simulink model "test08"  (R2021a)
settings: Solver=VariableStepAuto  StartTime=0.0  StopTime=10  RelTol=1e-3
values from neighbouring files (symbols this model uses):
  crop_params = crop_p    [test08_script.m]
  x0_crop = crop_ic    [test08_script.m]
libraries: HORTISIM x15
(part 1 of 2)
settings Model: Creator=djoroya  LastModifiedBy=djoroya
settings DebuggingCC: UnconnectedInputMsg=none  UnconnectedOutputMsg=none  UnconnectedLineMsg=none

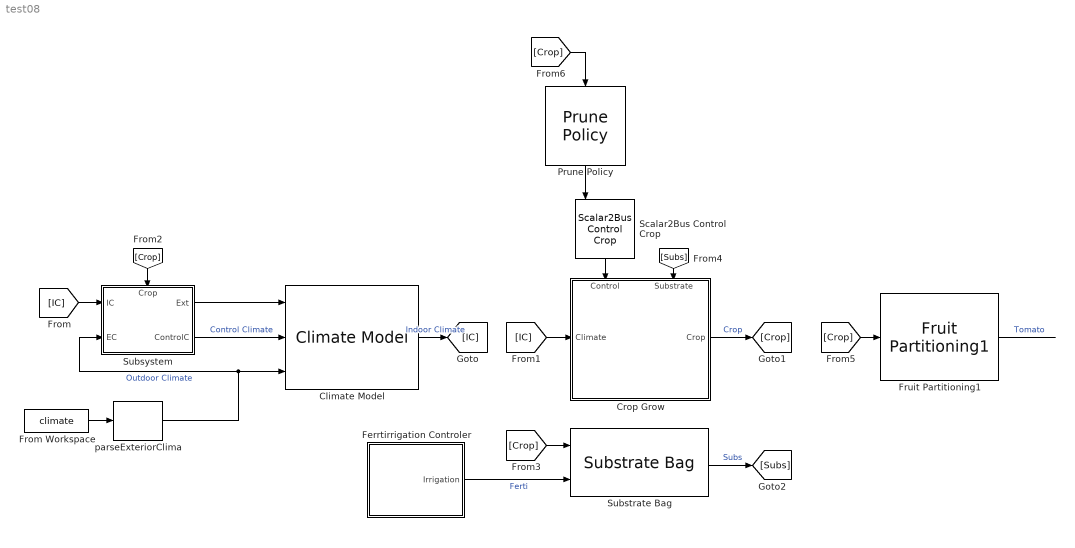
== system test08 ==
  Climate Model : HORTISIM/Climate/Models/Climate Model  params=params  x0=cic
      settings: SourceProductName=Horti Simulator
      mask Display: image('$imagefile'); % Use "Edit Image" on toolstrip to change.
  Crop Grow : Subsystem  AncestorBlock=HORTISIM/Horticulture/Models/Crop Grow  mask{params=crop_params, x0=x0_crop}
      settings: PortSchema="{\"entries\":[{\"content\":{\"sides\":[{\"content\":{\"connectorIds\":[\"In1\"]},\"type\":\"ConnectorPlacement.EquallySpacedRectSide\",\"uuid\":\"7d52d4c6-bc72-40ae-ba7a-fef791f60555\"},{\"content\":{\"connectorIds\":[\"Out1\"],\"side\":\"RIGHT\"},\"type\":\"ConnectorPlacement.EquallySpacedRectSide\",\"uuid\":\"3a9c2840-361d-4677-a7cc-c5f954b33f07\"},{\"content\":{\"connectorIds\":[\"In2\",\"In3\"],\"side\":\"TOP\"},\"type\":\"ConnectorPlacement.EquallySpacedRectSide\",\"uuid\":\"4fc8b0ee-86a8-4f1e-9fcc-25f95949aa32\"},{\"content\":{\"connectorIds\":[],\"side\":\"BOTTOM\"},\"type\":\"ConnectorPlacement.EquallySpacedRectSide\",\"uuid\":\"254dc665-acaf-49d5-9184-a028de083de6\"}]},\"type\":\"ConnectorPlacement.EquallySpacedConnector\",\"uuid\":\"4a2a8912-594b-41a4-9c04-2b6ae0329b55\"}],\"packageUris\":[\"http://schema.mathworks.com/mf0/Connector/R2020b\"],\"version\":\"1.0\"}"
      mask Display: image('$imagefile'); % Use "Edit Image" on toolstrip to change.
  Ferrtirrigation Controler : Subsystem  AncestorBlock="HORTISIM/Horticulture/Controls/Ferrtirrigation  Controler"
      mask Display: image('$imagefile'); % Use "Edit Image" on toolstrip to change.
  From Workspace : FromWorkspace  VariableName=climate
  Fruit Partitioning1 : HORTISIM/Horticulture/Models/Fruit Partitioning1  x0=x0_fruit  params=params_fruit
      settings: SourceProductName=Horti Simulator
      mask Display: image('tomato.png'); % Use "Edit Image" on toolstrip to change.
  Prune Policy : HORTISIM/Horticulture/Controls/Prune Policy  SystemSampleTime=-1  VariantActivationTime=update diagram  Latency=0  AutoFrameSizeCalculation=off
      settings: SourceProductName=Horti Simulator
      mask Display: image('$imagefile'); % Use "Edit Image" on toolstrip to change.
  Scalar2Bus Control Crop : HORTISIM/Other  Functions/Scalar2Bus Control Crop  SystemSampleTime=-1  VariantActivationTime=update diagram  Latency=0  AutoFrameSizeCalculation=off
      settings: SourceProductName=Horti Simulator
  Substrate Bag : HORTISIM/Horticulture/Models/Substrate Bag  x0=x0_substrate  params=substrate_params
      settings: SourceProductName=Horti Simulator
      mask Display: image('substrate.png'); % Use "Edit Image" on toolstrip to change.
  Subsystem : Subsystem
      settings: PortSchema="{\"entries\":[{\"content\":{\"sides\":[{\"content\":{\"connectorIds\":[\"In1\",\"In2\"]},\"type\":\"ConnectorPlacement.EquallySpacedRectSide\",\"uuid\":\"05a20284-31f0-4954-ac42-b08c051c723b\"},{\"content\":{\"connectorIds\":[\"Out1\",\"Out2\"],\"side\":\"RIGHT\"},\"type\":\"ConnectorPlacement.EquallySpacedRectSide\",\"uuid\":\"7e4ab434-6629-473e-82a5-f81f17f0ab6e\"},{\"content\":{\"connectorIds\":[\"In3\"],\"side\":\"TOP\"},\"type\":\"ConnectorPlacement.EquallySpacedRectSide\",\"uuid\":\"2ea64524-8947-456a-a977-2c05776eabaa\"}]},\"type\":\"ConnectorPlacement.EquallySpacedConnector\",\"uuid\":\"6035ded9-300f-4f3c-adde-f9d2e7ea6cf9\"}],\"packageUris\":[\"http://schema.mathworks.com/mf0/Connector/R2020b\"],\"version\":\"1.0\"}"
  parseExteriorClima : HORTISIM/Other  Functions/parseExteriorClima  SystemSampleTime=-1  VariantActivationTime=update diagram  Latency=0  AutoFrameSizeCalculation=off
      settings: SourceProductName=Horti Simulator
  wires:
  From Workspace/1 -> parseExteriorClima/1
  parseExteriorClima/1 -> Climate Model/3, Subsystem/2(EC)  "Outdoor Climate"
  Climate Model/1 -> [IC]  "Indoor Climate"
  Subsystem/2(ControlC) -> Climate Model/2  "Control Climate"
  [IC] -> Subsystem/1(IC)
  Subsystem/1(Ext) -> Climate Model/1
  [IC] -> Crop Grow/1(Climate)
  Crop Grow/1(Crop) -> [Crop]  "Crop"
  [Crop] -> Subsystem/3(Crop)
  [Crop] -> Substrate Bag/1
  Substrate Bag/1 -> [Subs]  "Subs"
  [Subs] -> Crop Grow/3(Substrate)
  Ferrtirrigation Controler/1(Irrigation) -> Substrate Bag/2  "Ferti"
  [Crop] -> Fruit Partitioning1/1
  Fruit Partitioning1/1 -> ?  "Tomato"
  Scalar2Bus Control Crop/1 -> Crop Grow/2(Control)
  Prune Policy/1 -> Scalar2Bus Control Crop/1
  [Crop] -> Prune Policy/1

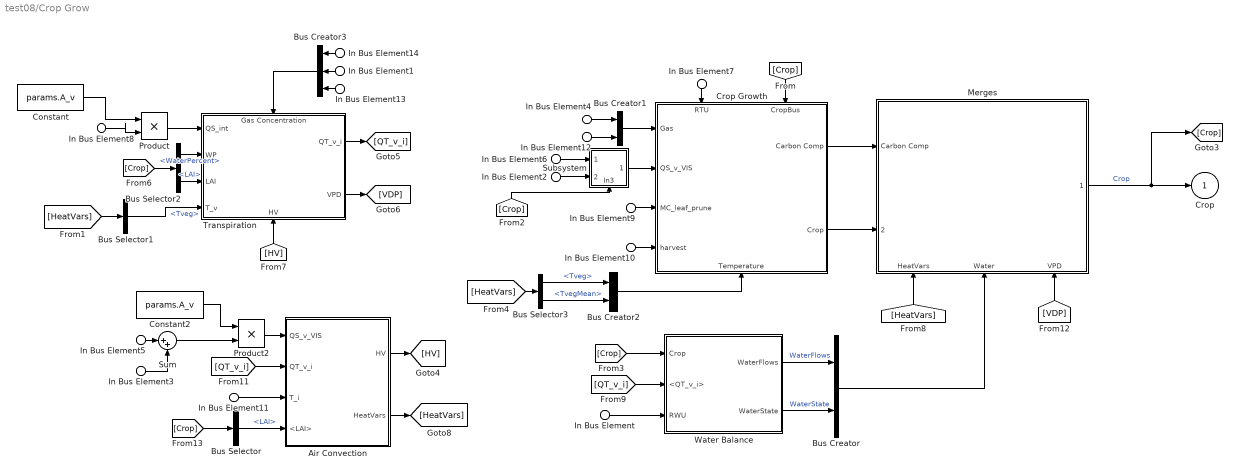
== system test08/Crop Grow ==
  In Bus Element8 : Inport  PortName=Climate  Element=QS.R_int
  In Bus Element3 : Inport  PortName=Climate  Element=QS.R_int
  In Bus Element2 : Inport  PortName=Climate  Element=QS.R_int
  In Bus Element11 : Inport  PortName=Climate  Element=Temp.Tair
  In Bus Element4 : Inport  PortName=Climate  Element=Gas.C_c
  In Bus Element12 : Inport  PortName=Climate  Element=Gas.rho_i
  In Bus Element13 : Inport  PortName=Climate  Element=Gas.rho_i
  In Bus Element1 : Inport  PortName=Climate  Element=Gas.C_c_ppm
  In Bus Element14 : Inport  PortName=Climate  Element=Gas.C_w
  In Bus Element9 : Inport  Port=2  PortName=Control  Element=Prune
  In Bus Element5 : Inport  Port=2  PortName=Control  Element=Artificial Rad
  In Bus Element6 : Inport  Port=2  PortName=Control  Element=Artificial Rad
  In Bus Element10 : Inport  Port=2  PortName=Control  Element=Harvest
  In Bus Element : Inport  Port=3  PortName=Substrate  Element=Uptake.Water
  In Bus Element7 : Inport  Port=3  PortName=Substrate  Element=Uptake.Nutrients
  Air Convection : Subsystem
  Bus Creator : BusCreator  Inputs=2
  Bus Creator1 : BusCreator  Inputs=2
  Bus Creator2 : BusCreator  Inputs=2
  Bus Creator3 : BusCreator  Inputs=3
  Bus Selector : BusSelector  OutputSignals=LAI
  Bus Selector1 : BusSelector  OutputSignals=Tveg
  Bus Selector2 : BusSelector  OutputSignals=WaterPercent,LAI
  Bus Selector3 : BusSelector  OutputSignals=Tveg,TvegMean
  Constant : Constant  Value=params.A_v
  Constant2 : Constant  Value=params.A_v
  Crop Growth : Subsystem
      settings: PortSchema="{\"entries\":[{\"content\":{\"sides\":[{\"content\":{\"connectorIds\":[\"In1\",\"In2\",\"In3\",\"In4\"]},\"type\":\"ConnectorPlacement.EquallySpacedRectSide\",\"uuid\":\"e694206d-cf53-43ea-b790-8b83ac78aa3a\"},{\"content\":{\"connectorIds\":[\"Out1\",\"Out2\"],\"side\":\"RIGHT\"},\"type\":\"ConnectorPlacement.EquallySpacedRectSide\",\"uuid\":\"93817abb-865a-4529-a53b-9aa59cd1156c\"},{\"content\":{\"connectorIds\":[\"In5\",\"In6\"],\"side\":\"TOP\"},\"type\":\"ConnectorPlacement.EquallySpacedRectSide\",\"uuid\":\"edd59083-b991-4826-870e-7da3bc3e48d4\"},{\"content\":{\"connectorIds\":[\"In7\"],\"side\":\"BOTTOM\"},\"type\":\"ConnectorPlacement.EquallySpacedRectSide\",\"uuid\":\"aa2b3153-bf16-47ed-b19e-45b92f713263\"}]},\"type\":\"ConnectorPlacement.EquallySpacedConnector\",\"uuid\":\"72640b1e-82d8-4725-bb34-7435bfc9f969\"}],\"packageUris\":[\"http://schema.mathworks.com/mf0/Connector/R2020b\"],\"version\":\"1.0\"}"
  Merges : Subsystem
      settings: PortSchema="{\"entries\":[{\"content\":{\"sides\":[{\"content\":{\"connectorIds\":[\"In1\",\"In2\"]},\"type\":\"ConnectorPlacement.EquallySpacedRectSide\",\"uuid\":\"f4887da6-2928-4f39-8f5f-a84d343119b4\"},{\"content\":{\"connectorIds\":[\"Out1\"],\"side\":\"RIGHT\"},\"type\":\"ConnectorPlacement.EquallySpacedRectSide\",\"uuid\":\"0df0d8c4-f19c-45da-a42d-26f0e872c274\"},{\"content\":{\"connectorIds\":[],\"side\":\"TOP\"},\"type\":\"ConnectorPlacement.EquallySpacedRectSide\",\"uuid\":\"3b0cc3f6-1cfb-43ac-8908-74a7a76931e3\"},{\"content\":{\"connectorIds\":[\"In3\",\"In4\",\"In5\"],\"side\":\"BOTTOM\"},\"type\":\"ConnectorPlacement.EquallySpacedRectSide\",\"uuid\":\"7e6672ca-68aa-4c3f-955a-240d8575a2c6\"}]},\"type\":\"ConnectorPlacement.EquallySpacedConnector\",\"uuid\":\"a8299565-1b25-4490-849f-a8fa281592c1\"}],\"packageUris\":[\"http://schema.mathworks.com/mf0/Connector/R2020b\"],\"version\":\"1.0\"}"
  Product : Product
  Product2 : Product
  Subsystem : Subsystem
      settings: PortSchema="{\"entries\":[{\"content\":{\"sides\":[{\"content\":{\"connectorIds\":[\"In1\",\"In2\"]},\"type\":\"ConnectorPlacement.EquallySpacedRectSide\",\"uuid\":\"c9e251e2-f19d-4856-b15c-3b9f1eb64f83\"},{\"content\":{\"connectorIds\":[\"Out1\"],\"side\":\"RIGHT\"},\"type\":\"ConnectorPlacement.EquallySpacedRectSide\",\"uuid\":\"10734817-c937-42fb-8ae5-9505620c6f0f\"},{\"content\":{\"connectorIds\":[],\"side\":\"TOP\"},\"type\":\"ConnectorPlacement.EquallySpacedRectSide\",\"uuid\":\"8c056440-d8bf-4ff4-85aa-0f6a5eb7f23f\"},{\"content\":{\"connectorIds\":[\"In3\"],\"side\":\"BOTTOM\"},\"type\":\"ConnectorPlacement.EquallySpacedRectSide\",\"uuid\":\"dd07dcd8-5298-4126-bdbb-0b047f66f0f4\"}]},\"type\":\"ConnectorPlacement.EquallySpacedConnector\",\"uuid\":\"13e72cfa-9d8f-4756-adac-f24fb0238c2a\"}],\"packageUris\":[\"http://schema.mathworks.com/mf0/Connector/R2020b\"],\"version\":\"1.0\"}"
  Sum : Sum  Inputs=|++
  Transpiration : Subsystem
      settings: PortSchema="{\"entries\":[{\"content\":{\"sides\":[{\"content\":{\"connectorIds\":[\"In1\",\"In2\",\"In3\",\"In4\"]},\"type\":\"ConnectorPlacement.EquallySpacedRectSide\",\"uuid\":\"d6bbd0cc-329a-44d5-b58b-a93078f7e5d1\"},{\"content\":{\"connectorIds\":[\"Out1\",\"Out2\"],\"side\":\"RIGHT\"},\"type\":\"ConnectorPlacement.EquallySpacedRectSide\",\"uuid\":\"249abf44-6c9b-4b00-a2f9-2043ee582e13\"},{\"content\":{\"connectorIds\":[\"In5\"],\"side\":\"TOP\"},\"type\":\"ConnectorPlacement.EquallySpacedRectSide\",\"uuid\":\"efa2d349-63e9-4701-9d30-a0c2adbee945\"},{\"content\":{\"connectorIds\":[\"In6\"],\"side\":\"BOTTOM\"},\"type\":\"ConnectorPlacement.EquallySpacedRectSide\",\"uuid\":\"decf1794-1744-434d-adf6-c7060d48f04b\"}]},\"type\":\"ConnectorPlacement.EquallySpacedConnector\",\"uuid\":\"1e3e15aa-c080-4684-9da5-24f03928e17f\"}],\"packageUris\":[\"http://schema.mathworks.com/mf0/Connector/R2020b\"],\"version\":\"1.0\"}"
  Water Balance : Subsystem
  Crop : Outport
  wires:
  [Crop] -> Subsystem/3(In3)
  In Bus Element10/1 -> Crop Growth/4(harvest)
  In Bus Element/1 -> Water Balance/3(RWU)
  Bus Selector3/1 -> Bus Creator2/1  "<Tveg>"
  [HeatVars] -> Bus Selector3/1
  [HeatVars] -> Bus Selector1/1
  Bus Creator/1 -> Merges/4(Water)
  Water Balance/2(WaterState) -> Bus Creator/2  "WaterState"
  Water Balance/1(WaterFlows) -> Bus Creator/1  "WaterFlows"
  In Bus Element7/1 -> Crop Growth/5(RTU)
  Subsystem/1(Out1) -> Crop Growth/2(QS_v_VIS)
  In Bus Element2/1 -> Subsystem/2(In2)
  In Bus Element6/1 -> Subsystem/1(In1)
  Sum/1 -> Product2/2
  In Bus Element3/1 -> Sum/2
  In Bus Element5/1 -> Sum/1
  Constant2/1 -> Product2/1
  Product2/1 -> Air Convection/1(QS_v_VIS)
  Product/1 -> Transpiration/1(QS_int)
  In Bus Element8/1 -> Product/2
  Constant/1 -> Product/1
  In Bus Element13/1 -> Bus Creator3/3
  In Bus Element1/1 -> Bus Creator3/2
  In Bus Element14/1 -> Bus Creator3/1
  [Crop] -> Crop Growth/6(CropBus)
  Air Convection/2(HeatVars) -> [HeatVars]
  Air Convection/1(HV) -> [HV]
  Bus Selector/1 -> Air Convection/4(<LAI>)  "<LAI>"
  In Bus Element11/1 -> Air Convection/3(T_i)
  [QT_v_i] -> Air Convection/2(QT_v_i)
  [QT_v_i] -> Water Balance/2(<QT_v_i>)
  [Crop] -> Water Balance/1(Crop)
  Crop Growth/2(Crop) -> Merges/2(" ")
  Crop Growth/1("Carbon Comp   ") -> Merges/1("Carbon Comp   ")
  Bus Creator2/1 -> Crop Growth/7(Temperature)
  In Bus Element9/1 -> Crop Growth/3(MC_leaf_prune)
  Bus Creator1/1 -> Crop Growth/1(Gas)
  [HeatVars] -> Merges/3(HeatVars)
  Bus Selector1/1 -> Transpiration/4(T_v)  "<Tveg>"
  [Crop] -> Bus Selector/1
  [VDP] -> Merges/5(VPD)
  Transpiration/2(VPD) -> [VDP]
  Transpiration/1(QT_v_i) -> [QT_v_i]
  Bus Selector2/2 -> Transpiration/3(LAI)  "<LAI>"
  [Crop] -> Bus Selector2/1
  Bus Selector2/1 -> Transpiration/2(WP)  "<WaterPercent>"
  Bus Creator3/1 -> Transpiration/5(Gas Concentration)
  [HV] -> Transpiration/6(HV)
  Bus Selector3/2 -> Bus Creator2/2  "<TvegMean>"
  In Bus Element12/1 -> Bus Creator1/2
  In Bus Element4/1 -> Bus Creator1/1
  Merges/1("    ") -> [Crop], Crop/1  "Crop"

== system test08/Ferrtirrigation Controler ==
  note: $kg\{H_2O\}/(s\cdot plant)$
  Bus Creator : BusCreator  Inputs=3  OutDataTypeStr=Bus: FLOW  NonVirtualBus=on
  Irrigation Controler : Subsystem
  "[Kelvin]" : Constant  Value=273.15 + 10
  kg/m^3 : Constant  Value=0.1 +zeros(8,1)
  Irrigation : Outport
  wires:
  kg/m^3/1 -> Bus Creator/3  "X"
  Irrigation Controler/1(Irrigation) -> Bus Creator/1  "f"
  "[Kelvin]"/1 -> Bus Creator/2  "T"
  Bus Creator/1 -> Irrigation/1

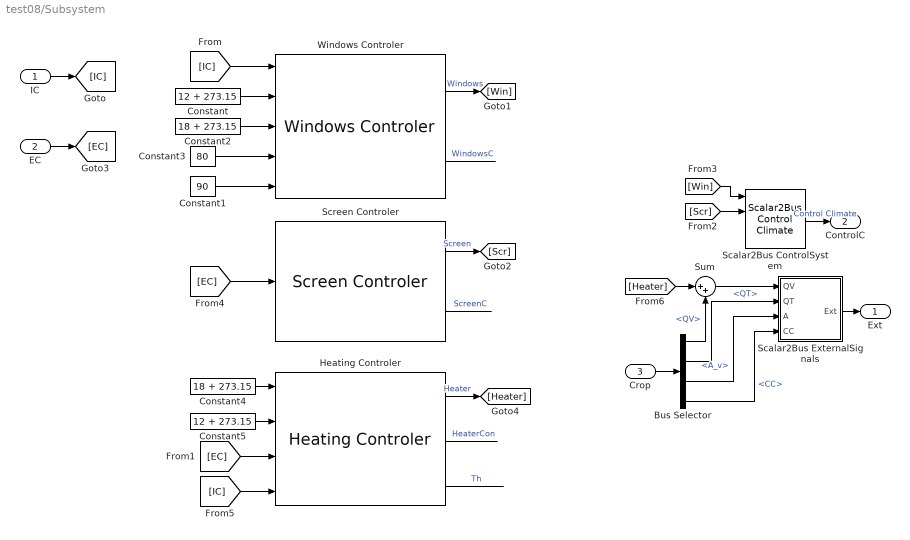
== system test08/Subsystem ==
  IC : Inport
  EC : Inport  Port=2
  Crop : Inport  Port=3
  Bus Selector : BusSelector  OutputSignals=HeatVars.QV,HeatVars.QT,A_v,CC
  Constant : Constant  Value=12 + 273.15
  Constant1 : Constant  Value=90
  Constant2 : Constant  Value=18 + 273.15
  Constant3 : Constant  Value=80
  Constant4 : Constant  Value=18 + 273.15
  Constant5 : Constant  Value=12 + 273.15
  Heating Controler : HORTISIM/Climate/Controls/Heating Controler  params=heat_p  x0=heat_ic
      settings: SourceProductName=Horti Simulator
  Scalar2Bus ControlSystem : HORTISIM/Other  Functions/Scalar2Bus  Control Climate  SystemSampleTime=-1  VariantActivationTime=update diagram  Latency=0  AutoFrameSizeCalculation=off
      settings: SourceProductName=Horti Simulator
  Scalar2Bus ExternalSignals : Subsystem
  Screen Controler : HORTISIM/Climate/Controls/Screen Controler  params=scr_p
      settings: SourceProductName=Horti Simulator
  Sum : Sum  Inputs=|++
  Windows Controler : HORTISIM/Climate/Controls/Windows Controler  params=win_p
      settings: SourceProductName=Horti Simulator
  Ext : Outport
  ControlC : Outport  Port=2
  wires:
  Constant2/1 -> Windows Controler/3
  Constant3/1 -> Windows Controler/4
  Windows Controler/2 -> ?  "WindowsC"
  Constant1/1 -> Windows Controler/5
  Constant/1 -> Windows Controler/2
  IC/1 -> [IC]
  [IC] -> Windows Controler/1
  Windows Controler/1 -> [Win]  "Windows"
  Screen Controler/1 -> [Scr]  "Screen"
  [Scr] -> Scalar2Bus ControlSystem/2
  [Win] -> Scalar2Bus ControlSystem/1
  Scalar2Bus ControlSystem/1 -> ControlC/1  "Control Climate"
  EC/1 -> [EC]
  [EC] -> Screen Controler/1
  Screen Controler/2 -> ?  "ScreenC"
  [EC] -> Heating Controler/3
  [IC] -> Heating Controler/4
  Constant4/1 -> Heating Controler/1
  Constant5/1 -> Heating Controler/2
  Heating Controler/1 -> [Heater]  "Heater"
  Scalar2Bus ExternalSignals/1(Ext) -> Ext/1
  Heating Controler/3 -> ?  "Th"
  Heating Controler/2 -> ?  "HeaterCon"
  Crop/1 -> Bus Selector/1
  Bus Selector/2 -> Scalar2Bus ExternalSignals/2(QT)  "<QT>"
  [Heater] -> Sum/1
  Sum/1 -> Scalar2Bus ExternalSignals/1(QV)
  Bus Selector/1 -> Sum/2  "<QV>"
  Bus Selector/3 -> Scalar2Bus ExternalSignals/3(A)  "<A_v>"
  Bus Selector/4 -> Scalar2Bus ExternalSignals/4(CC)  "<CC>"

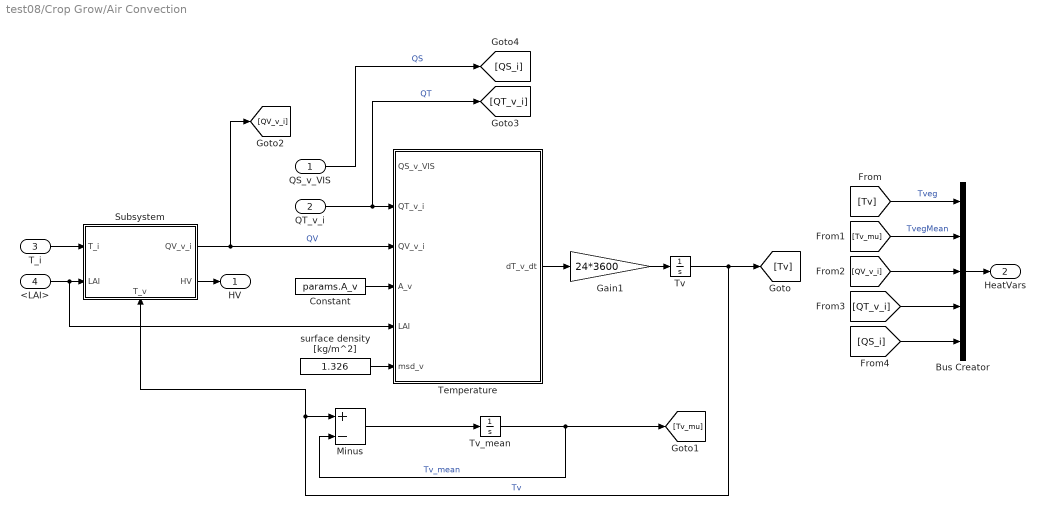
== system test08/Crop Grow/Air Convection ==
  QS_v_VIS : Inport
  QT_v_i : Inport  Port=2
  T_i : Inport  Port=3
  <LAI> : Inport  Port=4
  " Temperature" : MATLAB Function  TreatAsAtomicUnit=on
  Bus Creator : BusCreator  Inputs=5
  Constant : Constant  Value=params.A_v
  Gain1 : Gain  Gain=24*3600
  Minus : Sum  Inputs=+-
  Subsystem : Subsystem
      settings: PortSchema="{\"entries\":[{\"content\":{\"sides\":[{\"content\":{\"connectorIds\":[\"In1\",\"In2\"]},\"type\":\"ConnectorPlacement.EquallySpacedRectSide\",\"uuid\":\"4a223777-4148-4e71-aff8-25d93471e208\"},{\"content\":{\"connectorIds\":[\"Out1\",\"Out2\"],\"side\":\"RIGHT\"},\"type\":\"ConnectorPlacement.EquallySpacedRectSide\",\"uuid\":\"f67a472e-d82a-4194-8a1d-cf4d17d79652\"},{\"content\":{\"connectorIds\":[],\"side\":\"TOP\"},\"type\":\"ConnectorPlacement.EquallySpacedRectSide\",\"uuid\":\"dc13fded-a670-4e66-896d-6b985aeea447\"},{\"content\":{\"connectorIds\":[\"In3\"],\"side\":\"BOTTOM\"},\"type\":\"ConnectorPlacement.EquallySpacedRectSide\",\"uuid\":\"546dc1d6-9e48-4e4a-b9dc-c8e8ff8af02b\"}]},\"type\":\"ConnectorPlacement.EquallySpacedConnector\",\"uuid\":\"dd1fea49-cd8b-49b4-879c-c05a742382b3\"}],\"packageUris\":[\"http://schema.mathworks.com/mf0/Connector/R2020b\"],\"version\":\"1.0\"}"
  Tv : Integrator  InitialCondition=x0.Tv  AbsoluteTolerance=0.01
  Tv_mean : Integrator  InitialCondition=x0.Tv  AbsoluteTolerance=1e-3
  surface density [kg/m^2] : Constant  Value=1.326
  HV : Outport
  HeatVars : Outport  Port=2
  wires:
  Bus Creator/1 -> HeatVars/1
  [QS_i] -> Bus Creator/5
  [QT_v_i] -> Bus Creator/4
  [QV_v_i] -> Bus Creator/3
  [Tv_mu] -> Bus Creator/2  "TvegMean"
  [Tv] -> Bus Creator/1  "Tveg"
  QT_v_i/1 -> " Temperature"/2(QT_v_i), [QT_v_i]  "QT"
  QS_v_VIS/1 -> [QS_i]  "QS"
  Subsystem/1(QV_v_i) -> " Temperature"/3(QV_v_i), [QV_v_i]  "QV"
  Tv/1 -> Subsystem/3(T_v), Minus/1, [Tv]  "Tv"
  Minus/1 -> Tv_mean/1
  Tv_mean/1 -> Minus/2, [Tv_mu]  "Tv_mean"
  T_i/1 -> Subsystem/1(T_i)
  Subsystem/2(HV) -> HV/1
  <LAI>/1 -> " Temperature"/5(LAI), Subsystem/2(LAI)
  Constant/1 -> " Temperature"/4(A_v)
  surface density [kg/m^2]/1 -> " Temperature"/6(msd_v)
  " Temperature"/1(dT_v_dt) -> Gain1/1
  Gain1/1 -> Tv/1

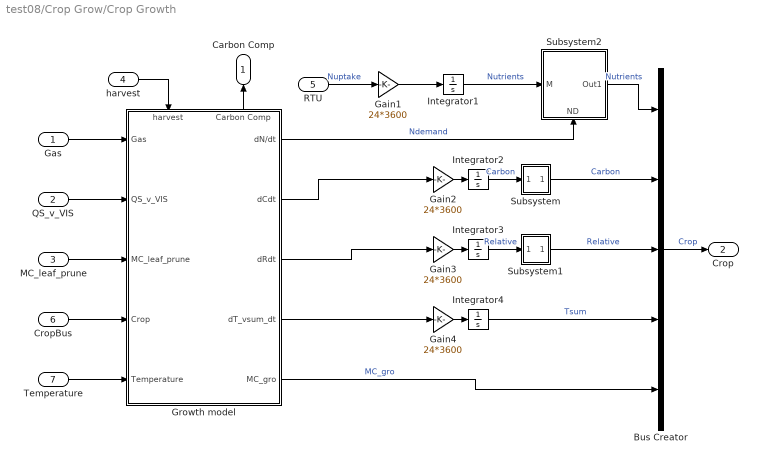
== system test08/Crop Grow/Crop Growth ==
  Gas : Inport
  QS_v_VIS : Inport  Port=2
  MC_leaf_prune : Inport  Port=3
  harvest : Inport  Port=4
  RTU : Inport  Port=5
  CropBus : Inport  Port=6
  Temperature : Inport  Port=7
  Bus Creator : BusCreator  Inputs=5
  Gain{1..4} (4 alike) : Gain  Gain=24*3600
  Growth model : Subsystem
      settings: PortSchema="{\"entries\":[{\"content\":{\"sides\":[{\"content\":{\"connectorIds\":[\"In1\",\"In2\",\"In3\",\"In4\",\"In5\"]},\"type\":\"ConnectorPlacement.EquallySpacedRectSide\",\"uuid\":\"524d3e03-5719-41db-bf49-dcf5dd5869ab\"},{\"content\":{\"connectorIds\":[\"Out1\",\"Out2\",\"Out3\",\"Out4\",\"Out5\"],\"side\":\"RIGHT\"},\"type\":\"ConnectorPlacement.EquallySpacedRectSide\",\"uuid\":\"b6ee0c40-6a76-4355-a893-3d13d29f29ea\"},{\"content\":{\"connectorIds\":[\"In6\",\"Out6\"],\"side\":\"TOP\"},\"type\":\"ConnectorPlacement.EquallySpacedRectSide\",\"uuid\":\"3cb45a24-0889-4a9a-ac04-e1ca208b77ae\"}]},\"type\":\"ConnectorPlacement.EquallySpacedConnector\",\"uuid\":\"fab17374-053c-4d8a-b11b-d7cd69978ad8\"}],\"packageUris\":[\"http://schema.mathworks.com/mf0/Connector/R2020b\"],\"version\":\"1.0\"}"
  Integrator1 : Integrator  InitialCondition=x0.N  AbsoluteTolerance=1e-4
  Integrator2 : Integrator  InitialCondition=x0.C  AbsoluteTolerance=1e-4
  Integrator3 : Integrator  InitialCondition=x0.R  AbsoluteTolerance=1e-9
  Integrator4 : Integrator  InitialCondition=x0.Tsum
  Subsystem : Subsystem
  Subsystem1 : Subsystem
  Subsystem2 : Subsystem
      settings: PortSchema="{\"entries\":[{\"content\":{\"sides\":[{\"content\":{\"connectorIds\":[\"In1\"]},\"type\":\"ConnectorPlacement.EquallySpacedRectSide\",\"uuid\":\"1f0226fa-6d14-4434-a5d5-098a94c6aa33\"},{\"content\":{\"connectorIds\":[\"Out1\"],\"side\":\"RIGHT\"},\"type\":\"ConnectorPlacement.EquallySpacedRectSide\",\"uuid\":\"12e08114-9d71-45f9-bd21-e03815fbba92\"},{\"content\":{\"connectorIds\":[],\"side\":\"TOP\"},\"type\":\"ConnectorPlacement.EquallySpacedRectSide\",\"uuid\":\"f70b570c-09d2-427a-8272-34c6eabee9a4\"},{\"content\":{\"connectorIds\":[\"In2\"],\"side\":\"BOTTOM\"},\"type\":\"ConnectorPlacement.EquallySpacedRectSide\",\"uuid\":\"db0772f6-92fe-46fe-85e5-ff48d92542ad\"}]},\"type\":\"ConnectorPlacement.EquallySpacedConnector\",\"uuid\":\"23ce1bc9-4d09-4c56-8e1c-5e49b0ef0462\"}],\"packageUris\":[\"http://schema.mathworks.com/mf0/Connector/R2020b\"],\"version\":\"1.0\"}"
  "Carbon Comp   " : Outport
  Crop : Outport  Port=2
  wires:
  harvest/1 -> Growth model/6(harvest)
  Growth model/1(dN/dt) -> Subsystem2/2(ND)  "Ndemand"
  Subsystem2/1(Out1) -> Bus Creator/1  "Nutrients"
  Integrator1/1 -> Subsystem2/1(M)  "Nutrients"
  RTU/1 -> Gain1/1  "Nuptake"
  Gain1/1 -> Integrator1/1
  Subsystem1/1(Out1) -> Bus Creator/3  "Relative"
  Integrator3/1 -> Subsystem1/1(In1)  "Relative"
  Integrator2/1 -> Subsystem/1(In1)  "Carbon"
  Subsystem/1(Out1) -> Bus Creator/2  "Carbon"
  Growth model/5(MC_gro) -> Bus Creator/5  "MC_gro"
  Temperature/1 -> Growth model/5(Temperature)
  CropBus/1 -> Growth model/4(Crop)
  Gain2/1 -> Integrator2/1
  QS_v_VIS/1 -> Growth model/2(QS_v_VIS)
  Growth model/2(dCdt) -> Gain2/1
  Growth model/4(dT_vsum_dt) -> Gain4/1
  Gain4/1 -> Integrator4/1
  Gain3/1 -> Integrator3/1
  Gas/1 -> Growth model/1(Gas)
  Growth model/3(dRdt) -> Gain3/1
  Integrator4/1 -> Bus Creator/4  "Tsum"
  MC_leaf_prune/1 -> Growth model/3(MC_leaf_prune)
  Growth model/6("Carbon Comp   ") -> "Carbon Comp   "/1
  Bus Creator/1 -> Crop/1  "Crop"

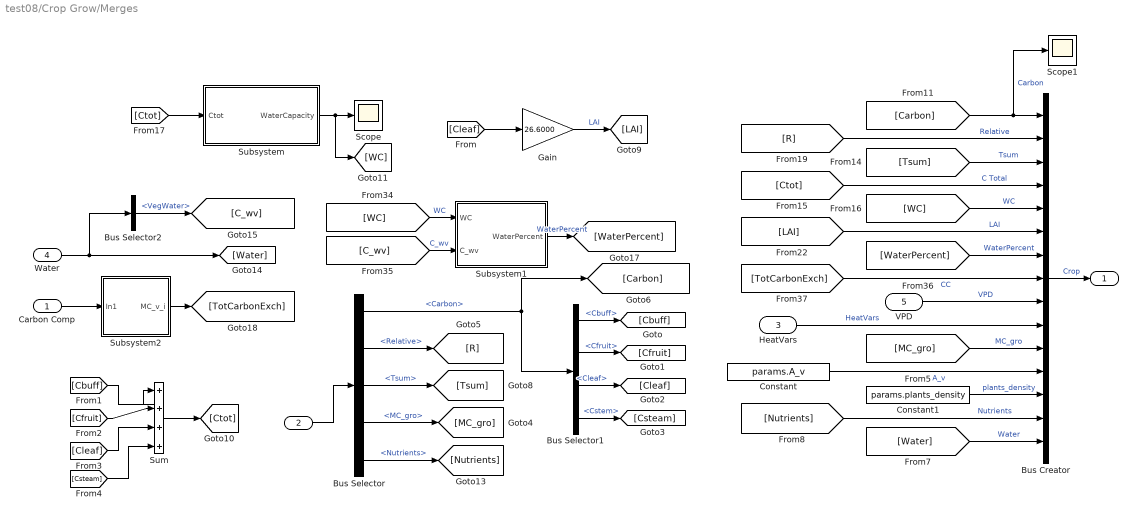
== system test08/Crop Grow/Merges ==
  "Carbon Comp   " : Inport
  " " : Inport  Port=2
  HeatVars : Inport  Port=3
  Water : Inport  Port=4
  VPD : Inport  Port=5
  Bus Creator : BusCreator  Inputs=15
  Bus Selector : BusSelector  OutputSignals=Carbon,Relative,Tsum,MC_gro,Nutrients
  Bus Selector1 : BusSelector  OutputSignals=Cbuff,Cfruit,Cleaf,Cstem
  Bus Selector2 : BusSelector  OutputSignals=WaterState.VegWater
  Constant : Constant  Value=params.A_v
  Constant1 : Constant  Value=params.plants_density
  Gain : Gain  Gain=26.6000
  Scope : Scope
  Scope1 : Scope
  Subsystem : Subsystem
  Subsystem1 : Subsystem
  Subsystem2 : Subsystem
  Sum : Sum  Inputs=|++++
  "    " : Outport
  wires:
  [Nutrients] -> Bus Creator/14  "Nutrients"
  Bus Selector/5 -> [Nutrients]  "<Nutrients>"
  Constant1/1 -> Bus Creator/13  "plants_density"
  [Ctot] -> Bus Creator/4  "C Total"
  Subsystem2/1(MC_v_i) -> [TotCarbonExch]
  [C_wv] -> Subsystem1/2(C_wv)  "C_wv"
  Bus Selector2/1 -> [C_wv]  "<VegWater>"
  Bus Selector/2 -> [R]  "<Relative>"
  Bus Selector1/2 -> [Cfruit]  "<Cfruit>"
  "Carbon Comp   "/1 -> Subsystem2/1(In1)
  Bus Selector/3 -> [Tsum]  "<Tsum>"
  [Carbon] -> Bus Creator/1, Scope1/1  "Carbon"
  [Water] -> Bus Creator/15  "Water"
  [WaterPercent] -> Bus Creator/7  "WaterPercent"
  Constant/1 -> Bus Creator/12  "A_v"
  [Csteam] -> Sum/4
  HeatVars/1 -> Bus Creator/10  "HeatVars"
  [MC_gro] -> Bus Creator/11  "MC_gro"
  Bus Selector/4 -> [MC_gro]  "<MC_gro>"
  [WC] -> Bus Creator/5  "WC"
  VPD/1 -> Bus Creator/9  "VPD"
  [TotCarbonExch] -> Bus Creator/8  "CC"
  Subsystem1/1(WaterPercent) -> [WaterPercent]  "WaterPercent"
  [WC] -> Subsystem1/1(WC)  "WC"
  Bus Selector1/4 -> [Csteam]  "<Cstem>"
  Bus Creator/1 -> "    "/1  "Crop"
  Bus Selector1/3 -> [Cleaf]  "<Cleaf>"
  Bus Selector1/1 -> [Cbuff]  "<Cbuff>"
  " "/1 -> Bus Selector/1
  [R] -> Bus Creator/2  "Relative"
  [LAI] -> Bus Creator/6  "LAI"
  [Tsum] -> Bus Creator/3  "Tsum"
  Water/1 -> [Water], Bus Selector2/1
  Bus Selector/1 -> [Carbon], Bus Selector1/1  "<Carbon>"
  Sum/1 -> [Ctot]
  [Cleaf] -> Sum/3
  [Cfruit] -> Sum/2
  [Cbuff] -> Sum/1
  [Ctot] -> Subsystem/1(Ctot)
  Subsystem/1(WaterCapacity) -> Scope/1, [WC]
  Gain/1 -> [LAI]  "LAI"
  [Cleaf] -> Gain/1

== system test08/Crop Grow/Subsystem ==
  In1 : Inport
  In2 : Inport  Port=2
  In3 : Inport  Port=3
  Bus Selector : BusSelector  OutputSignals=LAI
  Constant1 : Constant  Value=params.A_v
  Gain : Gain  Gain=2
  Product1 : Product  Inputs=3
  Scope : Scope
  Scope1 : Scope
  Subsystem : Subsystem
  Subsystem1 : Subsystem
  Sum : Sum  Inputs=|++
  Sum1 : Sum  Inputs=|++
  Out1 : Outport
  wires:
  Gain/1 -> Out1/1
  Product1/1 -> Gain/1
  Sum/1 -> Product1/1, Scope1/1
  [a_v_fVIS] -> Sum/2
  [a_v_rVIS] -> Sum/1
  Subsystem1/1(Out1) -> [a_v_rVIS]
  Bus Selector/1 -> Subsystem/1(<LAI>), Subsystem1/1(<LAI>)  "<LAI>"
  Subsystem/1(Out1) -> [a_v_fVIS], Scope/1
  In3/1 -> Bus Selector/1
  Constant1/1 -> Product1/2
  In1/1 -> Sum1/1
  Sum1/1 -> Product1/3
  In2/1 -> Sum1/2

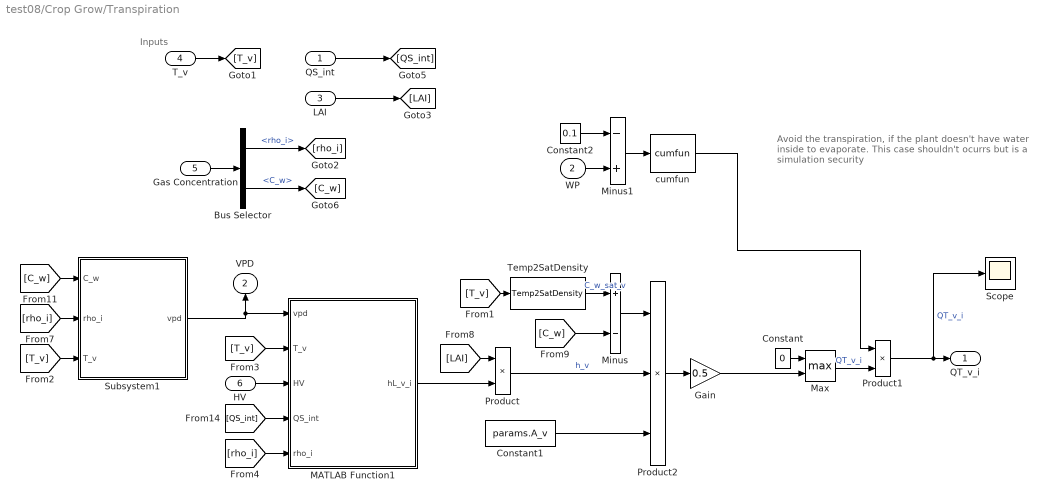
== system test08/Crop Grow/Transpiration ==
  note: Inputs
  note: Avoid the transpiration, if the plant
      |  doesn't have water inside to evaporate.
      | This case shouldn't ocurrs but is a simulation security
  QS_int : Inport
  WP : Inport  Port=2
  LAI : Inport  Port=3
  T_v : Inport  Port=4
  Gas Concentration : Inport  Port=5
  HV : Inport  Port=6
  Bus Selector : BusSelector  OutputSignals=rho_i,C_w
  Constant : Constant  Value=0
  Constant1 : Constant  Value=params.A_v
  Constant2 : Constant  Value=0.1
  Gain : Gain  Gain=0.5
  MATLAB Function1 : MATLAB Function  TreatAsAtomicUnit=on
  Max : MinMax  Function=max  Inputs=2
  Minus : Sum  Inputs=+-
  Minus1 : Sum  Inputs=-+
  Product : Product
  Product1 : Product
  Product2 : Product  Inputs=3
  Scope : Scope
  Subsystem1 : Subsystem
  Temp2SatDensity : HORTISIM/Other  Functions/Temp2SatDensity  SystemSampleTime=-1  VariantActivationTime=update diagram  Latency=0  AutoFrameSizeCalculation=off
      settings: SourceProductName=Horti Simulator
  cumfun : HORTISIM/Other  Functions/cumfun  SystemSampleTime=-1  VariantActivationTime=update diagram  Latency=0  AutoFrameSizeCalculation=off
      settings: SourceProductName=Horti Simulator
  QT_v_i : Outport
  VPD : Outport  Port=2
  wires:
  Minus1/1 -> cumfun/1
  cumfun/1 -> Product1/1
  Constant2/1 -> Minus1/1
  WP/1 -> Minus1/2
  [rho_i] -> MATLAB Function1/5(rho_i)
  [T_v] -> MATLAB Function1/2(T_v)
  Subsystem1/1(vpd) -> MATLAB Function1/1(vpd), VPD/1
  HV/1 -> MATLAB Function1/3(HV)
  [QS_int] -> MATLAB Function1/4(QS_int)
  MATLAB Function1/1(hL_v_i) -> Product/2
  [LAI] -> Product/1
  LAI/1 -> [LAI]
  [T_v] -> Subsystem1/3(T_v)
  [rho_i] -> Subsystem1/2(rho_i)
  [C_w] -> Subsystem1/1(C_w)
  Temp2SatDensity/1 -> Minus/1  "C_w_sat_v"
  [T_v] -> Temp2SatDensity/1
  Bus Selector/2 -> [C_w]  "<C_w>"
  Bus Selector/1 -> [rho_i]  "<rho_i>"
  Gas Concentration/1 -> Bus Selector/1
  QS_int/1 -> [QS_int]
  T_v/1 -> [T_v]
  [C_w] -> Minus/2
  Minus/1 -> Product2/1
  Product/1 -> Product2/2  "h_v"
  Constant1/1 -> Product2/3
  Product2/1 -> Gain/1
  Product1/1 -> QT_v_i/1, Scope/1  "QT_v_i"
  Constant/1 -> Max/1
  Max/1 -> Product1/2  "QT_v_i"
  Gain/1 -> Max/2

== system test08/Crop Grow/Water Balance ==
  note: $kg\{H_2O\}/(s\cdot m^2)$
  note: $kg\{H_2O\}/m^2$
  note: $kg\{H_2O\}/(s\cdot m^2)$
  Crop : Inport
  <QT_v_i> : Inport  Port=2
  RWU : Inport  Port=3
  Bus Selector : BusSelector  OutputSignals=WaterPercent,WC,A_v
  Divide : Product  Inputs=*//
  H_fg : Constant  Value=2437000
  Subsystem : Subsystem
  Subsystem1 : Subsystem
  Out Bus Element : Outport  PortName=WaterFlows  Element=WaterDemand
  Out Bus Element1 : Outport  PortName=WaterFlows  Element=WaterUptake
  Out Bus Element3 : Outport  PortName=WaterFlows  Element=MW_QT
  Out Bus Element6 : Outport  Port=2  PortName=WaterState  Element=VegWater
  wires:
  [MW_QT] -> Out Bus Element3/1
  Subsystem/1(C_wv) -> Out Bus Element6/1
  RWU/1 -> Subsystem/1(Real Water Uptake), [RWU]  "Real Water Uptake"
  Subsystem1/1(Out1) -> [DemandWater]
  Bus Selector/2 -> Subsystem1/2(<WC>)  "<WC>"
  Bus Selector/1 -> Subsystem1/1(<WaterPercent>)  "<WaterPercent>"
  Bus Selector/3 -> Divide/3  "<A_v>"
  [DemandWater] -> Out Bus Element/1
  [RWU] -> Out Bus Element1/1  "Real Water Uptake"
  Crop/1 -> Bus Selector/1
  H_fg/1 -> Divide/2
  <QT_v_i>/1 -> Divide/1
  Divide/1 -> Subsystem/2(Evapotranspiration), [MW_QT]  "Evapotranspiration"

== system test08/Ferrtirrigation Controler/Irrigation Controler ==
  note: $kg\{H_2O\}/(s\cdot m^2)$
  " " : Gain  Gain=5.6e-3
  Clock2 : Clock
  Constant1 : Constant  Value=24
  Gain4 : Gain  Gain=24
  If : If  IfExpression=(u1 > 6)&(u1<7)
  If Action Subsystem : Subsystem  TreatAsAtomicUnit=on
  If Action Subsystem1 : Subsystem  TreatAsAtomicUnit=on
  Merge : Merge
  Mod : Math  Operator=mod  SaturateOnIntegerOverflow=on
  Irrigation : Outport
  wires:
  Merge/1 -> " "/1
  If Action Subsystem1/1(Out1) -> Merge/2
  If Action Subsystem/1(Out1) -> Merge/1
  If/2 -> If Action Subsystem1/Action
  If/1 -> If Action Subsystem/Action
  Mod/1 -> If Action Subsystem/1(In1), If/1
  Gain4/1 -> Mod/1
  Clock2/1 -> Gain4/1
  Constant1/1 -> Mod/2
  " "/1 -> Irrigation/1

== system test08/Subsystem/Scalar2Bus ExternalSignals ==
  QV : Inport
  QT : Inport  Port=2
  A : Inport  Port=3
  CC : Inport  Port=4
  Bus Creator : BusCreator  Inputs=4
  Ext : Outport
  wires:
  QT/1 -> Bus Creator/2  "QT"
  QV/1 -> Bus Creator/1  "QV"
  A/1 -> Bus Creator/3  "A"
  CC/1 -> Bus Creator/4  "CC"
  Bus Creator/1 -> Ext/1

== system test08/Crop Grow/Air Convection/Subsystem ==
  T_i : Inport
  LAI : Inport  Port=2
  T_v : Inport  Port=3
  " characteristic leaf length [m]" : Constant  Value=0.5
  " characteristic leaf length [m]1" : Constant  Value=0.5
  Constant : Constant  Value=params.A_v
  Constant3 : Constant  Value=params.int_air_speed
  Convection1 : MATLAB Function  TreatAsAtomicUnit=on
  Raynols : MATLAB Function  TreatAsAtomicUnit=on
  QV_v_i : Outport
  HV : Outport  Port=2
  wires:
  [T_i] -> Convection1/1(T_i)
  [T_v] -> Convection1/3(T_v)
  [T_v] -> Raynols/2(T_v)
  [T_i] -> Raynols/1(T_i)
  T_v/1 -> [T_v]
  T_i/1 -> [T_i]
  Raynols/1(Nu) -> Convection1/2(Nu)
  LAI/1 -> Convection1/4(LAI)
  Convection1/1(QV_v_i) -> QV_v_i/1
  Convection1/2(HV) -> HV/1
  Constant/1 -> Convection1/5(A_v)
  " characteristic leaf length [m]"/1 -> Convection1/6(d_v)
  " characteristic leaf length [m]1"/1 -> Raynols/3(d_v)
  Constant3/1 -> Raynols/4(int_air_speed)

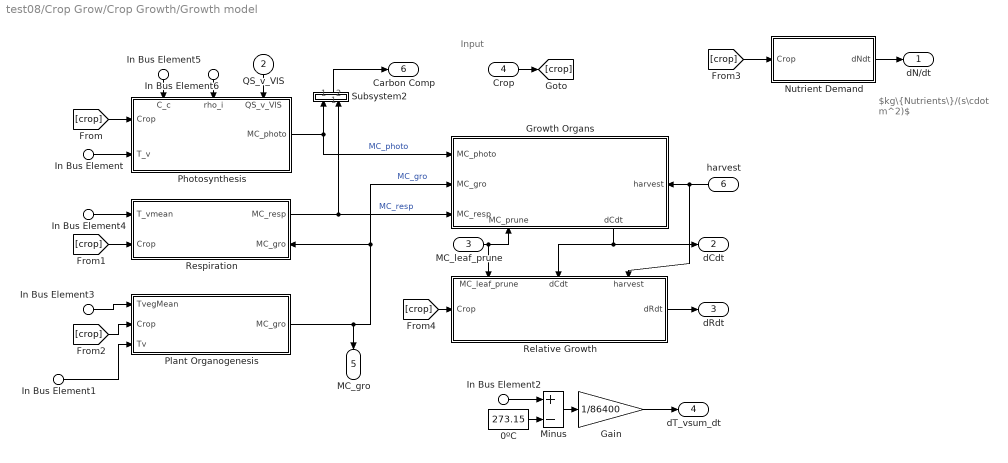
== system test08/Crop Grow/Crop Growth/Growth model ==
  note: $kg\{Nutrients\}/(s\cdot m^2)$
  note: Input
  In Bus Element5 : Inport  PortName=Gas  Element=C_c
  In Bus Element6 : Inport  PortName=Gas  Element=rho_i
  QS_v_VIS : Inport  Port=2
  MC_leaf_prune : Inport  Port=3
  Crop : Inport  Port=4
  In Bus Element : Inport  Port=5  PortName=Temperature  Element=Tveg
  In Bus Element1 : Inport  Port=5  PortName=Temperature  Element=Tveg
  In Bus Element2 : Inport  Port=5  PortName=Temperature  Element=TvegMean
  In Bus Element3 : Inport  Port=5  PortName=Temperature  Element=TvegMean
  In Bus Element4 : Inport  Port=5  PortName=Temperature  Element=TvegMean
  harvest : Inport  Port=6
  0ºC : Constant  Value=273.15
  Gain : Gain  Gain=1/86400
  Growth Organs : Subsystem
      settings: PortSchema="{\"entries\":[{\"content\":{\"sides\":[{\"content\":{\"connectorIds\":[\"In1\",\"In2\",\"In3\"]},\"type\":\"ConnectorPlacement.EquallySpacedRectSide\",\"uuid\":\"7ed23e67-f8bd-49ca-8750-2aec234a11ce\"},{\"content\":{\"connectorIds\":[\"In5\"],\"side\":\"RIGHT\"},\"type\":\"ConnectorPlacement.EquallySpacedRectSide\",\"uuid\":\"f57cc0dd-0cae-4ca4-a753-4e977147df3f\"},{\"content\":{\"connectorIds\":[],\"side\":\"TOP\"},\"type\":\"ConnectorPlacement.EquallySpacedRectSide\",\"uuid\":\"d3c6828c-1180-4cce-a803-c671dde62607\"},{\"content\":{\"connectorIds\":[\"In4\",\"Out1\"],\"side\":\"BOTTOM\"},\"type\":\"ConnectorPlacement.EquallySpacedRectSide\",\"uuid\":\"2964c671-ea65-49a5-9ed5-5f63619ae496\"}]},\"type\":\"ConnectorPlacement.EquallySpacedConnector\",\"uuid\":\"bc9ae77a-f1c5-46db-8e36-de23e641654c\"}],\"packageUris\":[\"http://schema.mathworks.com/mf0/Connector/R2020b\"],\"version\":\"1.0\"}"
  Minus : Sum  Inputs=+-
  Nutrient Demand : Subsystem
  Photosynthesis : Subsystem
      settings: PortSchema="{\"entries\":[{\"content\":{\"sides\":[{\"content\":{\"connectorIds\":[\"In1\",\"In2\"]},\"type\":\"ConnectorPlacement.EquallySpacedRectSide\",\"uuid\":\"5b7a12d1-e704-4d87-b94c-50c3f7e76c3e\"},{\"content\":{\"connectorIds\":[\"Out1\"],\"side\":\"RIGHT\"},\"type\":\"ConnectorPlacement.EquallySpacedRectSide\",\"uuid\":\"e5762904-c2a4-4288-9297-1f99c7dcb7bb\"},{\"content\":{\"connectorIds\":[\"In3\",\"In4\",\"In5\"],\"side\":\"TOP\"},\"type\":\"ConnectorPlacement.EquallySpacedRectSide\",\"uuid\":\"fedab1c2-3464-4f47-b4b1-20ddf7d17418\"}]},\"type\":\"ConnectorPlacement.EquallySpacedConnector\",\"uuid\":\"14a5d793-cc69-402c-a7d9-30d5c1b3824b\"}],\"packageUris\":[\"http://schema.mathworks.com/mf0/Connector/R2020b\"],\"version\":\"1.0\"}"
  "Plant Organogenesis " : Subsystem
  Relative Growth : Subsystem
      settings: PortSchema="{\"entries\":[{\"content\":{\"sides\":[{\"content\":{\"connectorIds\":[\"In1\"]},\"type\":\"ConnectorPlacement.EquallySpacedRectSide\",\"uuid\":\"3e921aa3-9028-45b3-8678-341874ae1dcc\"},{\"content\":{\"connectorIds\":[\"Out1\"],\"side\":\"RIGHT\"},\"type\":\"ConnectorPlacement.EquallySpacedRectSide\",\"uuid\":\"adeb12d0-e664-4860-aef8-c98149dc4c78\"},{\"content\":{\"connectorIds\":[\"In2\",\"In3\",\"In4\"],\"side\":\"TOP\"},\"type\":\"ConnectorPlacement.EquallySpacedRectSide\",\"uuid\":\"924e6078-7156-46d2-895a-2b088f75d5d0\"}]},\"type\":\"ConnectorPlacement.EquallySpacedConnector\",\"uuid\":\"ff0ec996-f79e-4632-97b2-da63dcaaf854\"}],\"packageUris\":[\"http://schema.mathworks.com/mf0/Connector/R2020b\"],\"version\":\"1.0\"}"
  Respiration : Subsystem
      settings: PortSchema="{\"entries\":[{\"content\":{\"sides\":[{\"content\":{\"connectorIds\":[\"In1\",\"In2\"]},\"type\":\"ConnectorPlacement.EquallySpacedRectSide\",\"uuid\":\"19bf8cd8-dcbb-428b-83dd-ef33216cf6f8\"},{\"content\":{\"connectorIds\":[\"Out1\",\"In3\"],\"side\":\"RIGHT\"},\"type\":\"ConnectorPlacement.EquallySpacedRectSide\",\"uuid\":\"fd2cf296-b399-40a0-bec1-532ab308bb18\"},{\"content\":{\"connectorIds\":[],\"side\":\"TOP\"},\"type\":\"ConnectorPlacement.EquallySpacedRectSide\",\"uuid\":\"43765028-08a6-45c9-8633-a0d1e070a8d0\"}]},\"type\":\"ConnectorPlacement.EquallySpacedConnector\",\"uuid\":\"d52fc605-80b9-4c52-aaab-d44015b38037\"}],\"packageUris\":[\"http://schema.mathworks.com/mf0/Connector/R2020b\"],\"version\":\"1.0\"}"
  Subsystem2 : Subsystem
  dN/dt : Outport
  dCdt : Outport  Port=2
  dRdt : Outport  Port=3
  dT_vsum_dt : Outport  Port=4
  MC_gro : Outport  Port=5
  "Carbon Comp   " : Outport  Port=6
  wires:
  In Bus Element1/1 -> "Plant Organogenesis "/3(Tv)
  harvest/1 -> Growth Organs/5(harvest), Relative Growth/4(harvest)
  [crop] -> Nutrient Demand/1(Crop)
  Growth Organs/1(dCdt) -> Relative Growth/3(dCdt), dCdt/1
  Nutrient Demand/1(dNdt) -> dN/dt/1
  In Bus Element6/1 -> Photosynthesis/4(rho_i)
  In Bus Element4/1 -> Respiration/1(T_vmean)
  [crop] -> Relative Growth/1(Crop)
  [crop] -> "Plant Organogenesis "/2(Crop)
  [crop] -> Respiration/2(Crop)
  [crop] -> Photosynthesis/1(Crop)
  Crop/1 -> [crop]
  In Bus Element3/1 -> "Plant Organogenesis "/1(TvegMean)
  In Bus Element/1 -> Photosynthesis/2(" T_v")
  MC_leaf_prune/1 -> Relative Growth/2(MC_leaf_prune), Growth Organs/4(MC_prune)
  "Plant Organogenesis "/1(MC_gro) -> Respiration/3(MC_gro), Growth Organs/2(MC_gro), MC_gro/1  "MC_gro"
  QS_v_VIS/1 -> Photosynthesis/5(QS_v_VIS)
  Photosynthesis/1(MC_photo) -> Growth Organs/1(MC_photo), Subsystem2/1(" ")  "MC_photo"
  In Bus Element5/1 -> Photosynthesis/3("C_c ")
  Gain/1 -> dT_vsum_dt/1
  Subsystem2/1("   ") -> "Carbon Comp   "/1
  Respiration/1(MC_resp) -> Growth Organs/3(MC_resp), Subsystem2/2("         ")  "MC_resp"
  Relative Growth/1(dRdt) -> dRdt/1
  In Bus Element2/1 -> Minus/1
  0ºC/1 -> Minus/2
  Minus/1 -> Gain/1

== system test08/Crop Grow/Crop Growth/Subsystem ==
  In1 : Inport
  Bus Creator : BusCreator  Inputs=4
  Demux : Demux
  Out1 : Outport
  wires:
  Bus Creator/1 -> Out1/1
  Demux/4 -> Bus Creator/4  "Cstem"
  Demux/3 -> Bus Creator/3  "Cleaf"
  Demux/2 -> Bus Creator/2  "Cfruit"
  Demux/1 -> Bus Creator/1  "Cbuff"
  In1/1 -> Demux/1

== system test08/Crop Grow/Crop Growth/Subsystem1 ==
  In1 : Inport
  Bus Creator : BusCreator  Inputs=3
  Demux : Demux  Outputs=3
  Out1 : Outport
  wires:
  Bus Creator/1 -> Out1/1
  Demux/3 -> Bus Creator/3  "Rstem"
  Demux/2 -> Bus Creator/2  "Rleaf"
  Demux/1 -> Bus Creator/1  "Rfruit"
  In1/1 -> Demux/1

== system test08/Crop Grow/Crop Growth/Subsystem2 ==
  M : Inport
  ND : Inport  Port=2
  Bus Creator : BusCreator  Inputs=2
  Out1 : Outport
  wires:
  Bus Creator/1 -> Out1/1
  M/1 -> Bus Creator/1  "Mass"
  ND/1 -> Bus Creator/2  "Demand"

== system test08/Crop Grow/Merges/Subsystem ==
  note: $kg\{H_2O\}/m^2$
  note: $kg\{H_2O\}/m^2$
  note: $kg\{H_2O\}/m^2$
  note: $kg\{H_2O\}/kg\{C\}$
  note: $kg\{C\}/m^2$
  Ctot : Inport
  Constant4 : Constant  Value=params.min_water_capacity
  Convertion Ratio : Subsystem
  Product : Product
  Sum : Sum  Inputs=|++
  WaterCapacity : Outport
  wires:
  Convertion Ratio/1(Out1) -> Product/2
  Sum/1 -> WaterCapacity/1
  Constant4/1 -> Sum/2
  Product/1 -> Sum/1
  Ctot/1 -> Product/1

== system test08/Crop Grow/Merges/Subsystem1 ==
  note: $kg\{H_2O\}/m^2$
  note: $kg\{H_2O\}/m^2$
  WC : Inport
  C_wv : Inport  Port=2
  Divide : Product  Inputs=*/
  WaterPercent : Outport
  wires:
  Divide/1 -> WaterPercent/1
  WC/1 -> Divide/2
  C_wv/1 -> Divide/1

== system test08/Crop Grow/Merges/Subsystem2 ==
  In1 : Inport
  " molar mass of CH2O [kg/mol]" : Constant  Value=0.03
  Bus Selector1 : BusSelector  OutputSignals=MC_i_buf,MC_buf_i,MC_fruit_i,MC_leaf_i,MC_stem_i
  Constant2 : Constant  Value=params.A_v
  Divide : Product  Inputs=*/**
  Sum1 : Sum  Inputs=|-++++
  molar mass of CO2 [kg/mol] : Constant  Value=0.044
  MC_v_i : Outport
  wires:
  Bus Selector1/1 -> Sum1/1  "<MC_i_buf>"
  Bus Selector1/5 -> Sum1/5  "<MC_stem_i>"
  " molar mass of CH2O [kg/mol]"/1 -> Divide/2
  Sum1/1 -> Divide/4
  Bus Selector1/2 -> Sum1/2  "<MC_buf_i>"
  Divide/1 -> MC_v_i/1  "MC_v_i"
  Constant2/1 -> Divide/3
  molar mass of CO2 [kg/mol]/1 -> Divide/1
  In1/1 -> Bus Selector1/1
  Bus Selector1/3 -> Sum1/3  "<MC_fruit_i>"
  Bus Selector1/4 -> Sum1/4  "<MC_leaf_i>"

== system test08/Crop Grow/Subsystem/Subsystem ==
  <LAI> : Inport
  Constant : Constant  Value=0.95
  Exp : Math  SaturateOnIntegerOverflow=on
  Gain : Gain  Gain=-1
  Gain1 : Gain  Gain=0.9
  Product : Product
  Sum : Sum  Inputs=|+-
  Visible diffuse extinction coefficient [-] : Constant  Value=0.85
  Out1 : Outport
  wires:
  Visible diffuse extinction coefficient [-]/1 -> Product/2
  Constant/1 -> Sum/1
  Gain/1 -> Exp/1
  Product/1 -> Gain/1
  Gain1/1 -> Sum/2
  Sum/1 -> Out1/1
  <LAI>/1 -> Product/1
  Exp/1 -> Gain1/1

== system test08/Crop Grow/Subsystem/Subsystem1 ==
  <LAI> : Inport
  Constant : Constant  Value=0.95
  Exp : Math  SaturateOnIntegerOverflow=on
  Gain : Gain  Gain=-1
  Gain1 : Gain  Gain=0.9
  Product : Product
  Sum : Sum  Inputs=|+-
  Visible diffuse extinction coefficient [-] : Constant  Value=0.5
  Out1 : Outport
  wires:
  Visible diffuse extinction coefficient [-]/1 -> Product/2
  Constant/1 -> Sum/1
  Gain/1 -> Exp/1
  Product/1 -> Gain/1
  Gain1/1 -> Sum/2
  Sum/1 -> Out1/1
  <LAI>/1 -> Product/1
  Exp/1 -> Gain1/1

== system test08/Crop Grow/Transpiration/Subsystem1 ==
  C_w : Inport
  rho_i : Inport  Port=2
  T_v : Inport  Port=3
  Constant : Constant  Value=0.622
  Divide : Product  Inputs=*/
  Divide1 : Product  Inputs=/*
  Divide2 : Product  Inputs=*/
  Divide3 : Product  Inputs=*/
  Minus : Sum  Inputs=-+
  Product : Product
  Sum : Sum  Inputs=|++
  Sum1 : Sum  Inputs=|++
  Temp2SatDensity : HORTISIM/Other  Functions/Temp2SatDensity  SystemSampleTime=-1  VariantActivationTime=update diagram  Latency=0  AutoFrameSizeCalculation=off
      settings: SourceProductName=Horti Simulator
  atm : Constant  Value=101300
  vpd : Outport
  wires:
  atm/1 -> Product/1
  Minus/1 -> Product/2
  Divide3/1 -> Minus/2
  Divide2/1 -> Minus/1
  Sum1/1 -> Divide3/2
  Sum/1 -> Divide2/2
  Divide/1 -> Sum/1, Divide2/1  "xa"
  Constant/1 -> Sum/2, Sum1/1
  Divide1/1 -> Sum1/2, Divide3/1  "xv"
  rho_i/1 -> Divide/2, Divide1/1
  Temp2SatDensity/1 -> Divide1/2
  T_v/1 -> Temp2SatDensity/1
  C_w/1 -> Divide/1
  Product/1 -> vpd/1  "vpd"

== system test08/Crop Grow/Water Balance/Subsystem ==
  Real Water Uptake : Inport
  Evapotranspiration : Inport  Port=2
  Gain8 : Gain  Gain=24*3600
  Sum : Sum  Inputs=|+-
  Water Content : Integrator  InitialCondition=x0.C_wv  AbsoluteTolerance=1e-3
  C_wv : Outport
  wires:
  Gain8/1 -> Water Content/1
  Real Water Uptake/1 -> Sum/1
  Water Content/1 -> C_wv/1  "C_wv"
  Sum/1 -> Gain8/1
  Evapotranspiration/1 -> Sum/2

== system test08/Crop Grow/Water Balance/Subsystem1 ==
  note: $1/s$
  note: $kg\{H_2O\}/m^2$
  <WaterPercent> : Inport
  <WC> : Inport  Port=2
  " " : Gain  Gain=5e-1
  Constant : Constant  Value=0.95
  Constant1 : Constant  Value=0
  Gain : Gain  Gain=1/100
  Max : MinMax  Function=max  Inputs=2
  Minus : Sum  Inputs=+-
  Product : Product
  Out1 : Outport
  wires:
  Gain/1 -> Product/1
  <WC>/1 -> Product/2
  Max/1 -> Out1/1
  Constant1/1 -> Max/2
  " "/1 -> Max/1
  Constant/1 -> Minus/1
  Product/1 -> " "/1
  Minus/1 -> Gain/1
  <WaterPercent>/1 -> Minus/2

== system test08/Ferrtirrigation Controler/Irrigation Controler/If Action Subsystem ==
  In1 : Inport
  Action Port : ActionPort  ActionPortLabel=if((u1 > 6)&(u1<7))
  Constant : Constant
  If : If  IfExpression=u1 > 0.5
  If Action Subsystem : Subsystem  TreatAsAtomicUnit=on
  If Action Subsystem1 : Subsystem  TreatAsAtomicUnit=on
  Merge : Merge
  Mod : Math  Operator=mod  SaturateOnIntegerOverflow=on
  Out1 : Outport
  wires:
  Merge/1 -> Out1/1
  If Action Subsystem1/1(Out1) -> Merge/2
  If Action Subsystem/1(Out1) -> Merge/1
  If/2 -> If Action Subsystem1/Action
  If/1 -> If Action Subsystem/Action
  Mod/1 -> If/1
  Constant/1 -> Mod/2
  In1/1 -> Mod/1

== system test08/Ferrtirrigation Controler/Irrigation Controler/If Action Subsystem1 ==
  Action Port : ActionPort  ActionPortLabel=else
  Constant : Constant  Value=0
  Out1 : Outport
  wires:
  Constant/1 -> Out1/1

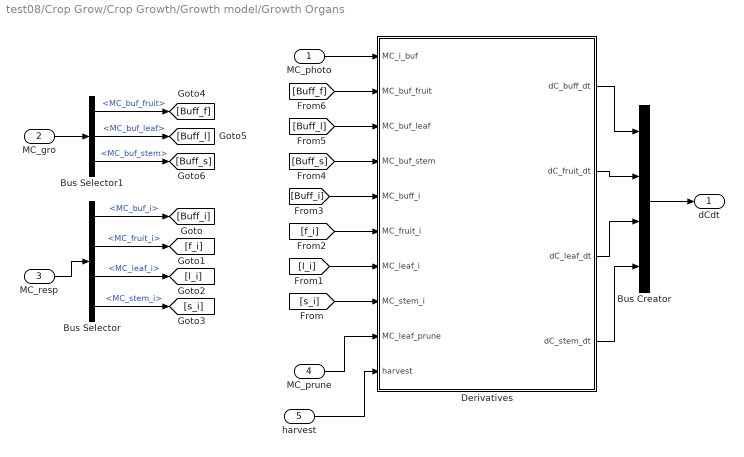
== system test08/Crop Grow/Crop Growth/Growth model/Growth Organs ==
  MC_photo : Inport
  MC_gro : Inport  Port=2
  MC_resp : Inport  Port=3
  MC_prune : Inport  Port=4
  harvest : Inport  Port=5
  Bus Creator : BusCreator  Inputs=4
  Bus Selector : BusSelector  OutputSignals=MC_buf_i,MC_fruit_i,MC_leaf_i,MC_stem_i
  Bus Selector1 : BusSelector  OutputSignals=MC_buf_fruit,MC_buf_leaf,MC_buf_stem
  Derivatives : MATLAB Function  TreatAsAtomicUnit=on
  dCdt : Outport
  wires:
  [Buff_f] -> Derivatives/2(MC_buf_fruit)
  [Buff_l] -> Derivatives/3(MC_buf_leaf)
  [Buff_s] -> Derivatives/4(MC_buf_stem)
  [Buff_i] -> Derivatives/5(MC_buff_i)
  [f_i] -> Derivatives/6(MC_fruit_i)
  [l_i] -> Derivatives/7(MC_leaf_i)
  [s_i] -> Derivatives/8(MC_stem_i)
  Bus Selector1/3 -> [Buff_s]  "<MC_buf_stem>"
  Bus Selector1/2 -> [Buff_l]  "<MC_buf_leaf>"
  Bus Selector1/1 -> [Buff_f]  "<MC_buf_fruit>"
  Bus Selector/3 -> [l_i]  "<MC_leaf_i>"
  Bus Selector/2 -> [f_i]  "<MC_fruit_i>"
  Bus Selector/4 -> [s_i]  "<MC_stem_i>"
  Bus Selector/1 -> [Buff_i]  "<MC_buf_i>"
  harvest/1 -> Derivatives/10(harvest)
  Derivatives/1(dC_buff_dt) -> Bus Creator/1
  MC_photo/1 -> Derivatives/1(MC_i_buf)
  MC_gro/1 -> Bus Selector1/1
  MC_resp/1 -> Bus Selector/1
  Bus Creator/1 -> dCdt/1
  Derivatives/4(dC_stem_dt) -> Bus Creator/4
  Derivatives/3(dC_leaf_dt) -> Bus Creator/3
  Derivatives/2(dC_fruit_dt) -> Bus Creator/2
  MC_prune/1 -> Derivatives/9(MC_leaf_prune)

== system test08/Crop Grow/Crop Growth/Growth model/Nutrient Demand ==
  note: $kg\{Nutrients\}/(s\cdot m^2)$
  Crop : Inport
  Bus Selector : BusSelector  OutputSignals=Carbon.Cfruit,Carbon.Cleaf,Carbon.Cstem,Nutrients.Mass
  Gain : Gain  Gain=params.Chi_nutrients
  Gain1 : Gain  Gain=1e-3
  Minus : Sum  Inputs=+-
  Sum of Elements1 : Sum  Inputs=+++
  dNdt : Outport
  wires:
  Minus/1 -> Gain1/1
  [chi_opt] -> Minus/1
  Gain/1 -> [chi_opt]
  Bus Selector/4 -> Minus/2  "<Mass>"
  Gain1/1 -> dNdt/1
  Sum of Elements1/1 -> Gain/1
  Bus Selector/1 -> Sum of Elements1/1  "<Cfruit>"
  Bus Selector/2 -> Sum of Elements1/2  "<Cleaf>"
  Bus Selector/3 -> Sum of Elements1/3  "<Cstem>"
  Crop/1 -> Bus Selector/1

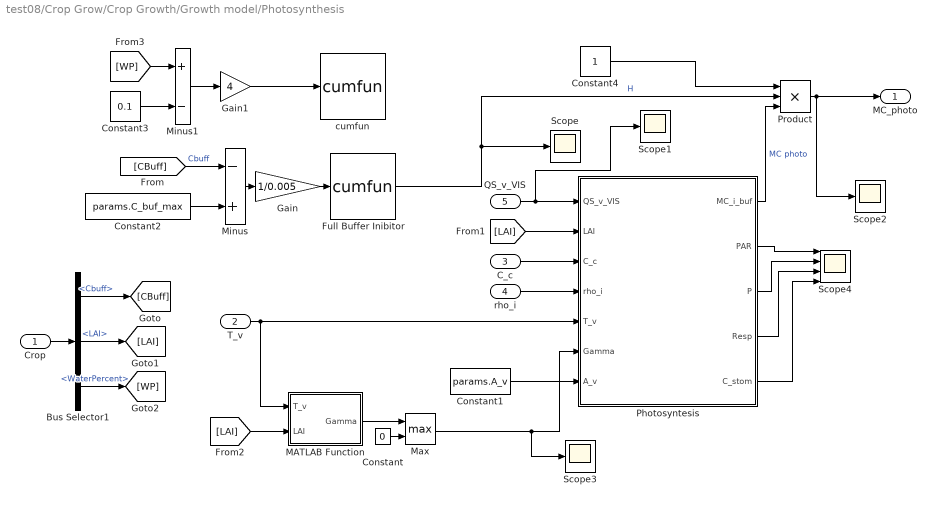
== system test08/Crop Grow/Crop Growth/Growth model/Photosynthesis ==
  Crop : Inport
  " T_v" : Inport  Port=2
  "C_c " : Inport  Port=3
  rho_i : Inport  Port=4
  QS_v_VIS : Inport  Port=5
  Bus Selector1 : BusSelector  OutputSignals=Carbon.Cbuff,LAI,WaterPercent
  Constant : Constant  Value=0
  Constant1 : Constant  Value=params.A_v
  Constant2 : Constant  Value=params.C_buf_max
  Constant3 : Constant  Value=0.1
  Constant4 : Constant
  Full Buffer Inibitor : HORTISIM/Other  Functions/cumfun  SystemSampleTime=-1  VariantActivationTime=update diagram  Latency=0  AutoFrameSizeCalculation=off
      settings: SourceProductName=Horti Simulator
  Gain : Gain  Gain=1/0.005
  Gain1 : Gain  Gain=4
  MATLAB Function : MATLAB Function  TreatAsAtomicUnit=on
  Max : MinMax  Function=max  Inputs=2
  Minus : Sum  Inputs=-+
  Minus1 : Sum  Inputs=+-
  Photosyntesis : MATLAB Function  TreatAsAtomicUnit=on
  Product : Product  Inputs=3
  Scope{,1..3} (4 alike) : Scope
  Scope4 : Scope  NumInputPorts=4
  cumfun : HORTISIM/Other  Functions/cumfun  SystemSampleTime=-1  VariantActivationTime=update diagram  Latency=0  AutoFrameSizeCalculation=off
      settings: SourceProductName=Horti Simulator
  MC_photo : Outport
  wires:
  Photosyntesis/5(C_stom) -> Scope4/4
  Photosyntesis/4(Resp) -> Scope4/3
  Photosyntesis/3(P) -> Scope4/2
  Photosyntesis/2(PAR) -> Scope4/1
  Gain1/1 -> cumfun/1
  Bus Selector1/1 -> [CBuff]  "<Cbuff>"
  [LAI] -> MATLAB Function/2(LAI)
  [LAI] -> Photosyntesis/2(LAI)
  Bus Selector1/2 -> [LAI]  "<LAI>"
  QS_v_VIS/1 -> Photosyntesis/1(QS_v_VIS), Scope1/1
  " T_v"/1 -> Photosyntesis/5(T_v), MATLAB Function/1(T_v)
  Crop/1 -> Bus Selector1/1
  Max/1 -> Photosyntesis/6(Gamma), Scope3/1
  Constant/1 -> Max/2
  MATLAB Function/1(Gamma) -> Max/1
  rho_i/1 -> Photosyntesis/4(rho_i)
  "C_c "/1 -> Photosyntesis/3(C_c)
  Constant1/1 -> Photosyntesis/7(A_v)
  Full Buffer Inibitor/1 -> Product/2, Scope/1  "H"
  Gain/1 -> Full Buffer Inibitor/1
  Minus/1 -> Gain/1
  Constant2/1 -> Minus/2
  [CBuff] -> Minus/1  "Cbuff"
  Bus Selector1/3 -> [WP]  "<WaterPercent>"
  [WP] -> Minus1/1
  Constant3/1 -> Minus1/2
  Minus1/1 -> Gain1/1
  Photosyntesis/1(MC_i_buf) -> Product/3  "MC photo"
  Product/1 -> MC_photo/1, Scope2/1
  Constant4/1 -> Product/1

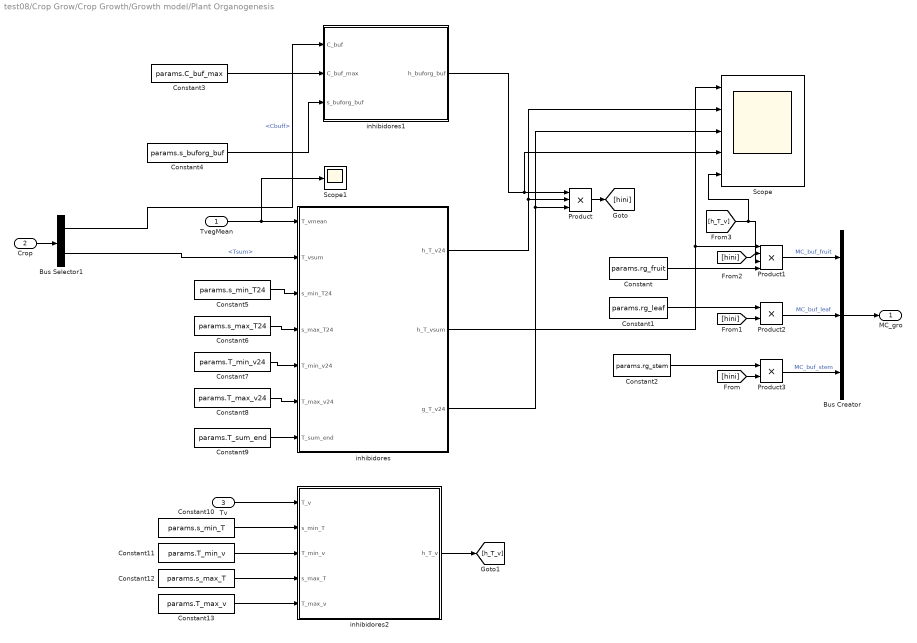
== system test08/Crop Grow/Crop Growth/Growth model/Plant Organogenesis  ==
  TvegMean : Inport
  Crop : Inport  Port=2
  Tv : Inport  Port=3
  Bus Creator : BusCreator  Inputs=3
  Bus Selector1 : BusSelector  OutputSignals=Carbon.Cbuff,Tsum
  Constant : Constant  Value=params.rg_fruit
  Constant1 : Constant  Value=params.rg_leaf
  Constant10 : Constant  Value=params.s_min_T
  Constant11 : Constant  Value=params.T_min_v
  Constant12 : Constant  Value=params.s_max_T
  Constant13 : Constant  Value=params.T_max_v
  Constant2 : Constant  Value=params.rg_stem
  Constant3 : Constant  Value=params.C_buf_max
  Constant4 : Constant  Value=params.s_buforg_buf
  Constant5 : Constant  Value=params.s_min_T24
  Constant6 : Constant  Value=params.s_max_T24
  Constant7 : Constant  Value=params.T_min_v24
  Constant8 : Constant  Value=params.T_max_v24
  Constant9 : Constant  Value=params.T_sum_end
  Product : Product  Inputs=3
  Product1 : Product  Inputs=4
  Product2 : Product
  Product3 : Product
  Scope : Scope  NumInputPorts=5
  Scope1 : Scope
  inhibidores : MATLAB Function  TreatAsAtomicUnit=on
  inhibidores1 : MATLAB Function  TreatAsAtomicUnit=on
  inhibidores2 : MATLAB Function  TreatAsAtomicUnit=on
  MC_gro : Outport
  wires:
  [h_T_v] -> Product1/3, Scope/5
  inhibidores2/1(h_T_v) -> [h_T_v]
  Constant13/1 -> inhibidores2/5(T_max_v)
  Constant12/1 -> inhibidores2/4(s_max_T)
  Constant11/1 -> inhibidores2/3(T_min_v)
  Constant10/1 -> inhibidores2/2(s_min_T)
  Tv/1 -> inhibidores2/1(T_v)
  Constant4/1 -> inhibidores1/3(s_buforg_buf)
  Bus Selector1/1 -> inhibidores1/1(C_buf)  "<Cbuff>"
  TvegMean/1 -> inhibidores/1(T_vmean), Scope1/1
  Bus Selector1/2 -> inhibidores/2(T_vsum)  "<Tsum>"
  Product3/1 -> Bus Creator/3  "MC_buf_stem"
  Product2/1 -> Bus Creator/2  "MC_buf_leaf"
  Product1/1 -> Bus Creator/1  "MC_buf_fruit"
  inhibidores/3(g_T_v24) -> Product/3, Scope/3
  inhibidores/1(h_T_v24) -> Product/2, Scope/2
  Bus Creator/1 -> MC_gro/1
  Crop/1 -> Bus Selector1/1
  Constant3/1 -> inhibidores1/2(C_buf_max)
  Constant5/1 -> inhibidores/3(s_min_T24)
  Constant6/1 -> inhibidores/4(s_max_T24)
  Constant7/1 -> inhibidores/5(T_min_v24)
  Constant8/1 -> inhibidores/6(T_max_v24)
  Constant9/1 -> inhibidores/7(T_sum_end)
  inhibidores1/1(h_buforg_buf) -> Product/1, Scope/4
  Constant/1 -> Product1/4
  inhibidores/2(h_T_vsum) -> Product1/1, Scope/1
  Constant1/1 -> Product2/1
  Constant2/1 -> Product3/1
  Product/1 -> [hini]
  [hini] -> Product3/2
  [hini] -> Product2/2
  [hini] -> Product1/2

== system test08/Crop Grow/Crop Growth/Growth model/Relative Growth ==
  Crop : Inport
  MC_leaf_prune : Inport  Port=2
  dCdt : Inport  Port=3
  harvest : Inport  Port=4
  Bus Selector : BusSelector  OutputSignals=Carbon.Cbuff,Carbon.Cfruit,Carbon.Cleaf,Relative.Rfruit,Relative.Rleaf,Relative.Rstem
  Bus Selector1 : BusSelector  OutputSignals=dC_fruit_dt,dC_fruit_dt,dC_fruit_dt
  Relative Growth : MATLAB Function  TreatAsAtomicUnit=on
  Vector Concatenate : Concatenate  NumInputs=3
  dRdt : Outport
  wires:
  harvest/1 -> Relative Growth/11(harvest)
  Bus Selector/1 -> Relative Growth/4(C_fruit)  "<Cbuff>"
  Bus Selector/2 -> Relative Growth/5(C_leaf)  "<Cfruit>"
  Bus Selector/3 -> Relative Growth/6(C_stem)  "<Cleaf>"
  Bus Selector/4 -> Relative Growth/7(R_fruit)  "<Rfruit>"
  Bus Selector/5 -> Relative Growth/8(R_leaf)  "<Rleaf>"
  Bus Selector/6 -> Relative Growth/9(R_stem)  "<Rstem>"
  Bus Selector1/3 -> Relative Growth/3(dC_stem_dt)  "<dC_fruit_dt>"
  Bus Selector1/1 -> Relative Growth/1(dC_fruit_dt)  "<dC_fruit_dt>"
  Bus Selector1/2 -> Relative Growth/2(dC_leaf_dt)  "<dC_fruit_dt>"
  dCdt/1 -> Bus Selector1/1
  Crop/1 -> Bus Selector/1
  Vector Concatenate/1 -> dRdt/1
  MC_leaf_prune/1 -> Relative Growth/10(MC_leaf_prune)
  Relative Growth/1(dR_fruit_dt) -> Vector Concatenate/1
  Relative Growth/3(dR_stem_dt) -> Vector Concatenate/3
  Relative Growth/2(dR_leaf_dt) -> Vector Concatenate/2
